simulink model "sistemaNonLineare"  (R2023b)
settings: Solver=VariableStepAuto  StartTime=0.0  StopTime=10.0  RelTol=1e-3
values from neighbouring files (symbols this model uses):
  C = [1, 0]    [C1_punto_3.m]    (also in CAT_C1 punti 1-2.m; CAT_C1_punti1_2.m; CAT_C1_punti3_4.m; progetto_C1.m)
  u_e = 9.81*m+k*x_1e    (= 199525)    [C1_punto_3.m]    (also in CAT_C1_punti3_4.m; progetto_C1.m)
  x_e = [x_1e;x_2e]    [C1_punto_3.m]    (also in CAT_C1_punti3_4.m; progetto_C1.m)
  ze = 0.35    [C1_punto_3.m]    (also in CAT_C1 punti 1-2.m; CAT_C1_punti1_2.m; CAT_C1_punti3_4.m; progetto_C1.m)
libraries: cstblocks x1
settings Model: Creator=Utente  LastModifiedBy=Utente

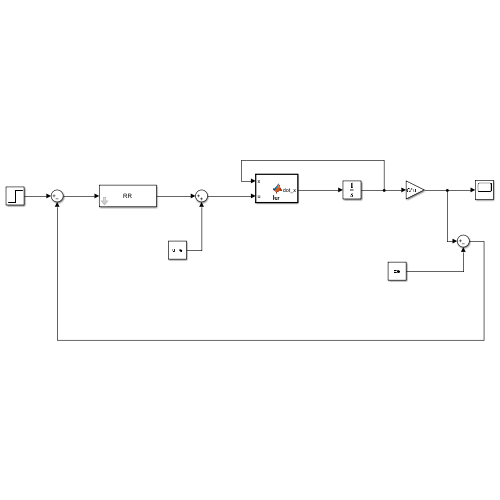
[thumbnail: Simulink's stored preview of the top-level diagram]
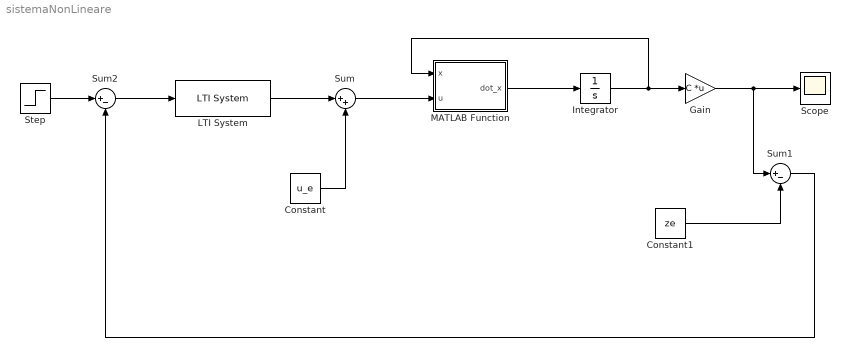
== system sistemaNonLineare ==
  Constant : Constant  Value=u_e
  Constant1 : Constant  Value=ze
  Gain : Gain  Gain=C  Multiplication=Matrix(K*u)
  Integrator : Integrator  InitialCondition=x_e
  LTI System : cstblocks/LTI System  sys=RR  IC=[]  PadeOrder=0
  MATLAB Function : MATLAB Function  TreatAsAtomicUnit=on
  Scope : Scope
  Step : Step  SampleTime=0
  Sum : Sum  Inputs=|++
  Sum1 : Sum  Inputs=|+-
  Sum2 : Sum  Inputs=|+-
  wires:
  LTI System/1 -> Sum/1
  Constant/1 -> Sum/2
  Sum/1 -> MATLAB Function/2(u)
  MATLAB Function/1(dot_x) -> Integrator/1
  Integrator/1 -> MATLAB Function/1(x), Gain/1
  Gain/1 -> Sum1/1, Scope/1
  Constant1/1 -> Sum1/2
  Step/1 -> Sum2/1
  Sum2/1 -> LTI System/1
  Sum1/1 -> Sum2/2

== matlab function sistemaNonLineare/MATLAB Function ==
  data: x input; u input; dot_x output
function dot_x = fcn(x,u)

m = 2500;       %% mass
b = 350;        %% smorzamento
k = 5*10^5;     %% cost. elastica lineare
n = 3;
g = 9.81;
beta = 0.1;

dot_x = zeros(2,1);

dot_x(1) = x(2);

dot_x(2) = -g - b*x(2)/m - k*x(1)/m  + beta/m * (x(2)^3 + n*x(2)*sin(n*x(2))^2) + u/m;
